simulink model "RoverTwinControl"  (R2024b)
settings: Solver=FixedStepDiscrete  StartTime=0.0  StopTime=inf  FixedStep=0.02  RelTol=1e-3
InitFcn:
  | rover_prepare_simulation
StopFcn:
  | rover_stop_simulation
undefined symbols (not defined in the file or in its folder): DiscIntNeverNeededParam
libraries: sim3dlib x4, sim3dphyssensorlib x1
settings Model: Creator=dinuk  LastModifiedBy=dinuk

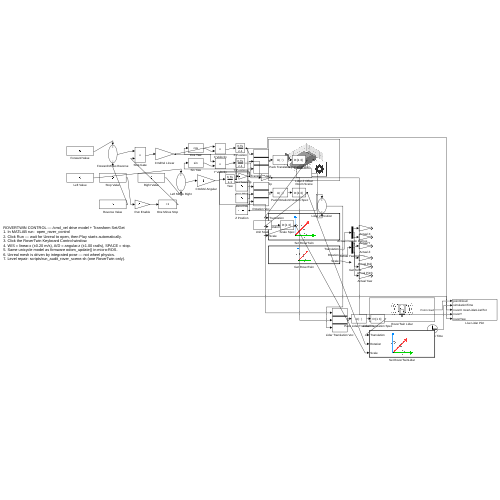
[thumbnail: Simulink's stored preview of the top-level diagram]
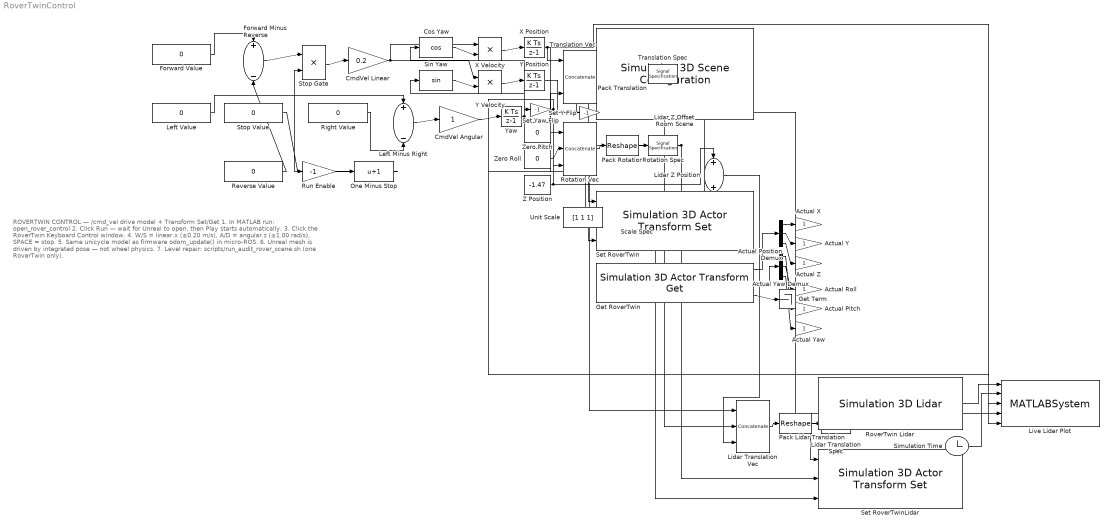
== system RoverTwinControl ==
  note: ROVERTWIN CONTROL — /cmd_vel drive model + Transform Set/Get
      | 1. In MATLAB run:  open_rover_control
      | 2. Click Run — wait for Unreal to open, then Play starts automatically.
      | 3. Click the RoverTwin Keyboard Control window.
      | 4. W/S = linear.x (±0.20 m/s), A/D = angular.z (±1.00 rad/s), SPACE = stop.
      | 5. Same unicycle model as firmware odom_update() in micro-ROS.
      | 6. Unreal mesh is driven by integrated pose — not wheel physics.
      | 7. Level repair: scripts/run_audit_rover_scene.sh (one RoverTwin only).
  Actual Pitch : Gain
  Actual Position Demux : Demux  Outputs=3
  Actual Roll : Gain
  Actual X : Gain
  Actual Y : Gain
  Actual Yaw : Gain
  Actual Yaw Demux : Demux  Outputs=3
  Actual Z : Gain
  CmdVel Angular : Gain
  CmdVel Linear : Gain  Gain=0.2
  Cos Yaw : Trigonometry  Operator=cos
  Forward Minus Reverse : Sum  Inputs=+-
  Forward Value : Constant  Value=0  OutDataTypeStr=double
  Get RoverTwin : sim3dlib/Simulation 3D Actor Transform Get  Priority=1  ActorTag=RoverTwin  NumberOfParts=1  CustNumOfParts=3  Ts=-1  aMode=aMode
  Get Term : Terminator
  Left Minus Right : Sum  Inputs=+-
  Left Value : Constant  Value=0  OutDataTypeStr=double
  Lidar Translation Spec : SignalSpecification  Dimensions=[1 3]
  Lidar Translation Vec : Concatenate  NumInputs=3  ConcatenateDimension=2
  Lidar Z Offset : Constant  Value=0.079
  Lidar Z Position : Sum
  Live Lidar Plot : MATLABSystem  System=roverLidarLivePlot  AxisLimit=8  PlotEvery=1  MaxPoints=4000  UdpPort=55221  UdpStaleSec=0.25  SimulateUsing=Interpreted execution
      mask Type: roverLidarLivePlot
      mask Display:
      | disp('roverLidarLivePlot');
      | port_label('input',1,'pointCloud');
      | port_label('input',2,'simulationTime');
      | port_label('input',3,'roverX');
      | port_label('input',4,'roverY');
      | port_label('input',5,'roverYaw');
  One Minus Stop : Bias  Bias=1  SaturateOnIntegerOverflow=off
  Pack Lidar Translation : Reshape  OutputDimensions=[1 3]
  Pack Rotation : Reshape  OutputDimensions=[1 3]
  Pack Translation : Reshape  OutputDimensions=[1 3]
  Reverse Value : Constant  Value=0  OutDataTypeStr=double
  Right Value : Constant  Value=0  OutDataTypeStr=double
  Room Scene : sim3dlib/Simulation 3D Scene Configuration  Priority=0  ProjectFormat=Unreal Editor  SceneDesc=Straight road  ProjectName=/home/dinuk/MATLAB/R2024b/toolbox/shared/sim3d_projects/automotive_project_linux/UE/LinuxNoEditor/VehicleSimulation.sh  ScenePath=/Game/Maps/MyRoom  UEProjPath=/tmp/RoverTwinUnrealProject/RoverTwin/RoverTwin.uproject  EnableOpenDRIVE=off  vehTagList="{\"Scene Origin\", \"RoverTwin\"}"  vehTag=Scene Origin  FreeCameraInitialTranslation=[1.25 0.8 4]  FreeCameraDefaultInitialTranslation=[-6, 0, 2]  FreeCameraInitialRotation=[-90, 0, 0]  FreeCameraDefaultInitialRotation=[0, -15, 0]  OpVisEn=off  Ts=0.02  EnableWindow=on  EnableRemoteAccess=off  EnableWeather=off  SunAzimuth=90  SunAltitude=40.0  EnableGeospatialSun=off  Latitude=0  Longitude=0  Date=2023-01-01  Time=10:30:00  GeoTimeZone=-5.0  SunDaylightSaving=off  wind=1  clouds=10  EnableVolumetricClouds=off  CloudCoverage=0  CloudAltitude=6  fog=0  rain=0  RaindropsEffect=off  SnowDensity=0  EnableGeospatial=off  UseTrueOrigin=off  OriginHeight=200  OriginLatitude=40.744652  OriginLongitude=-73.988864  MapStyle=Aerial  AdditionalAssetIDs=[]  UseAdvancedSunSky=off  SolarTime=11  TimeZone=-5  Day=21  Month=9  Year=2022  UseDaylightSavingTime=on  DSTStartDay=10  DSTStartMonth=3  DSTEndDay=3  DSTEndMonth=11  DSTSwitchHour=2  sensorTag=MainCamera1  sensorId=1  sensorName=MainCamera1  mountLoc=Origin  offsetFlag=off  tmountOffset=[0, 0, 0]  rmountOffset=[0, 0, 0]  HorizontalResolution=1280  VerticalResolution=720  HorizontalFOV=60  mountPoint=[0 0 0]  mountOrientation=[0 0 0]  aMode=3  ID=1  GeoTrigger=Inactive
      settings: LibrarySourceBlock=drivingsim3d/Simulation 3D Scene Configuration
  Rotation Spec : SignalSpecification  Dimensions=[1 3]
  Rotation Vec : Concatenate  NumInputs=3  ConcatenateDimension=2
  RoverTwin Lidar : sim3dphyssensorlib/Simulation 3D Lidar  Priority=1  sensorTag=RoverTwinLidar  sensorId=1  sensorName=RoverTwinLidar  vehTagList="{\"Scene Origin\", \"RoverTwin\"}"  vehTag=RoverTwin  mountLoc=Origin  offsetFlag=on  tmountOffset=[0, 0, 0]  rmountOffset=[0, 0, 0]  DetectionRange=8  RangeResolution=0.002  VerticalFOV=1  VerticalResolution=1  HorizontalFOV=360  HorizontalResolution=1  DistanceOutportEnabled=off  ReflectivityOutportEnabled=off  SemanticOutportEnabled=off  TransformOutportEnabled=off  SampleTime=0.1  mountPoint=[0 0 0]  mountOrientation=[0 0 0]  aMode=5  ID=1
      settings: LibrarySourceBlock=sl3dlib/Simulation 3D/Sensors/Simulation 3D Lidar
  Run Enable : Gain  Gain=-1
  Scale Spec : SignalSpecification  Dimensions=[1 3]
  Set RoverTwin : sim3dlib/Simulation 3D Actor Transform Set  Priority=-2  ActorTag=RoverTwin  NumberOfParts=1  CustNumOfParts=3  Translation=[1.25 0.8 -1.47]  Rotation=[0 0 0]  Scale=[1 1 1]  Ts=0.02  aMode=aMode
  Set RoverTwinLidar : sim3dlib/Simulation 3D Actor Transform Set  Priority=-1  ActorTag=RoverTwinLidar  NumberOfParts=1  CustNumOfParts=3  Translation=[1.25 0.8 -1.47]  Rotation=[0 0 0]  Scale=[1 1 1]  Ts=0.02  aMode=aMode
  Set Y Flip : Gain  Gain=-1
  Set Yaw Flip : Gain  Gain=-1
  Simulation Time : Clock
  Sin Yaw : Trigonometry
  Stop Gate : Product  Inputs=**
  Stop Value : Constant  Value=0  OutDataTypeStr=double
  Translation Spec : SignalSpecification  Dimensions=[1 3]
  Translation Vec : Concatenate  NumInputs=3  ConcatenateDimension=2
  Unit Scale : Constant  Value=[1 1 1]  VectorParams1D=off
  X Position : DiscreteIntegrator  InitialCondition=1.25  SampleTime=0.02  ICPrevOutput=DiscIntNeverNeededParam  ICPrevScaledInput=DiscIntNeverNeededParam
  X Velocity : Product
  Y Position : DiscreteIntegrator  InitialCondition=-0.8  SampleTime=0.02  ICPrevOutput=DiscIntNeverNeededParam  ICPrevScaledInput=DiscIntNeverNeededParam
  Y Velocity : Product
  Yaw : DiscreteIntegrator  SampleTime=0.02  ICPrevOutput=DiscIntNeverNeededParam  ICPrevScaledInput=DiscIntNeverNeededParam
  Z Position : Constant  Value=-1.47
  Zero Pitch : Constant  Value=0
  Zero Roll : Constant  Value=0
  wires:
  Get RoverTwin/3 -> Get Term/1
  RoverTwin Lidar/1 -> Live Lidar Plot/1
  Simulation Time/1 -> Live Lidar Plot/2
  Get RoverTwin/1 -> Actual Position Demux/1
  Get RoverTwin/2 -> Actual Yaw Demux/1
  Actual Position Demux/1 -> Actual X/1
  Actual Position Demux/2 -> Actual Y/1
  Actual Position Demux/3 -> Actual Z/1
  Actual Yaw Demux/1 -> Actual Pitch/1
  Actual Yaw Demux/2 -> Actual Roll/1
  Actual Yaw Demux/3 -> Actual Yaw/1
  Forward Value/1 -> Forward Minus Reverse/1
  Reverse Value/1 -> Forward Minus Reverse/2
  Left Value/1 -> Left Minus Right/1
  Right Value/1 -> Left Minus Right/2
  Stop Value/1 -> Run Enable/1
  Run Enable/1 -> One Minus Stop/1
  Forward Minus Reverse/1 -> Stop Gate/1
  One Minus Stop/1 -> Stop Gate/2
  Stop Gate/1 -> CmdVel Linear/1
  Left Minus Right/1 -> CmdVel Angular/1
  CmdVel Angular/1 -> Yaw/1
  Yaw/1 -> Cos Yaw/1, Sin Yaw/1, Set Yaw Flip/1
  CmdVel Linear/1 -> X Velocity/1, Y Velocity/1
  Cos Yaw/1 -> X Velocity/2
  Sin Yaw/1 -> Y Velocity/2
  X Velocity/1 -> X Position/1
  Y Velocity/1 -> Y Position/1
  X Position/1 -> Translation Vec/1, Lidar Translation Vec/1, Live Lidar Plot/3
  Y Position/1 -> Set Y Flip/1
  Set Y Flip/1 -> Translation Vec/2, Lidar Translation Vec/2, Live Lidar Plot/4
  Z Position/1 -> Translation Vec/3, Lidar Z Position/1
  Translation Vec/1 -> Pack Translation/1
  Pack Translation/1 -> Translation Spec/1
  Lidar Z Offset/1 -> Lidar Z Position/2
  Lidar Z Position/1 -> Lidar Translation Vec/3
  Lidar Translation Vec/1 -> Pack Lidar Translation/1
  Pack Lidar Translation/1 -> Lidar Translation Spec/1
  Zero Pitch/1 -> Rotation Vec/1
  Zero Roll/1 -> Rotation Vec/2
  Set Yaw Flip/1 -> Rotation Vec/3, Live Lidar Plot/5
  Rotation Vec/1 -> Pack Rotation/1
  Pack Rotation/1 -> Rotation Spec/1
  Unit Scale/1 -> Scale Spec/1
  Translation Spec/1 -> Set RoverTwin/1
  Rotation Spec/1 -> Set RoverTwin/2, Set RoverTwinLidar/2
  Scale Spec/1 -> Set RoverTwin/3, Set RoverTwinLidar/3
  Lidar Translation Spec/1 -> Set RoverTwinLidar/1
